simulink model "Flyback"  (R2018a)
settings: Solver=FixedStepDiscrete  StartTime=0.0  StopTime=stop_time  FixedStep=step_size  RelTol=1e-3
values from neighbouring files (symbols this model uses):
  Cf = 1e-4    (= 0.0001)    [sim_flyback.m]
  D = 0.4    [sim_flyback.m]
  f_s = 2e5    (= 200000)    [sim_flyback.m]
  R_L = 50    [sim_flyback.m]
  step_size = 1e-7    (= 1e-07)    [sim_flyback.m]
  Vd = 48    [sim_flyback.m]
libraries: powerlib x10, dspstat3 x3
settings Model: Creator=enes_  LastModifiedBy=enes_

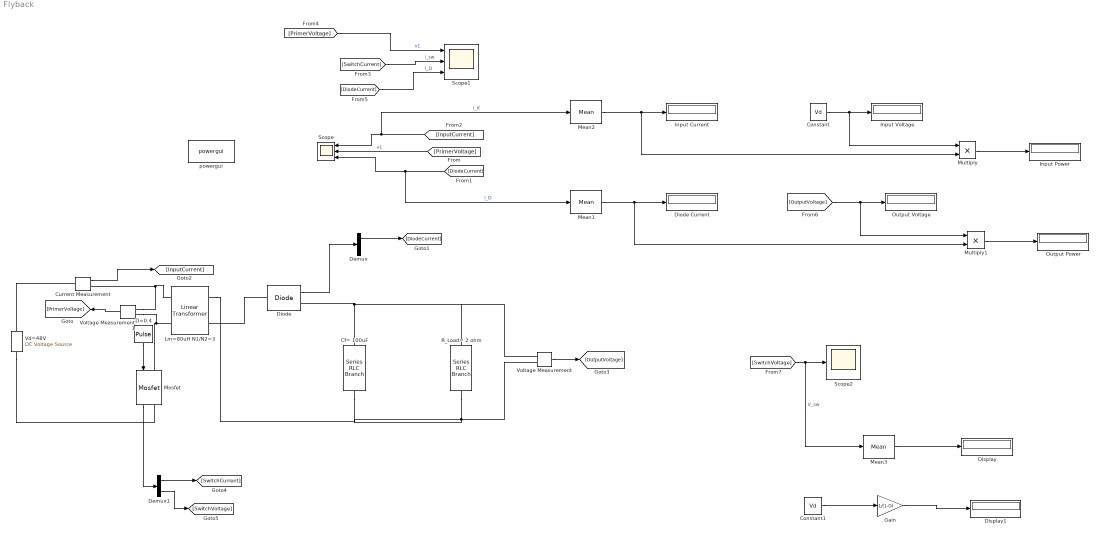
== system Flyback ==
  Cf= 100uF : powerlib/Elements/Series RLC Branch  LConnTagsString=__new0  RConnTagsString=__new0  BranchType=C  Resistance=1  Inductance=1e-3  SetiL0=off  InitialCurrent=0  Capacitance=Cf  Setx0=off  InitialVoltage=0  Measurements=None
  Constant : Constant  Value=Vd
  Constant1 : Constant  Value=Vd
  Current Measurement : powerlib/Measurements/Current Measurement  PhasorSimulation=off  OutputType=Complex  PSBequivalent=0
  D=0.4 : DiscretePulseGenerator  PulseType=Time based  Period=1/f_s  PulseWidth=100*D
  Demux : Demux  Outputs=2
  Demux1 : Demux  Outputs=2
  Diode : powerlib/Power Electronics/Diode  Ron=1e-8  Lon=0  Vf=0  IC=0  UseSnubber=0  Rs=500  Cs=250e-9  Measurements=on
  Diode Current : Display
  Display : Display
  Display1 : Display
  Gain : Gain  Gain=1/(1-D)
  Input Current : Display
  Input Power : Display
  Input Voltage : Display
  Lm=80uH N1/N2=3 : powerlib/Elements/Linear Transformer  UNITS=SI  NominalPower=[ 25 2e5 ]  winding1=[48 1e-8 1e-8 ]  winding2=[16 1e-8 1e-8]  ThreeWindings=off  winding3=[3.15e+05 0.7938 0.084225]  RmLm=[1e9 8e-5]  Measurements=All voltages and currents  DataType=on
  Mean1 : dspstat3/Mean  run=on  InputProcessing=Columns as channels (frame based)  reset_popup=None  directionMode=Each column  dimension=1  roiEnable=off  roiType=Rectangles  roiPortion=Entire ROI  roiOutput=Individual statistics for each ROI  roiFlag=off  roundingMode=Floor  overflowMode=off  outputDataTypeStr=Inherit: Same as accumulator  outputMin=[]  outputMax=[]  outputLastDataTypeStr=Inherit: Same as accumulator
  Mean2 : dspstat3/Mean  run=on  InputProcessing=Columns as channels (frame based)  reset_popup=None  directionMode=Each column  dimension=1  roiEnable=off  roiType=Rectangles  roiPortion=Entire ROI  roiOutput=Individual statistics for each ROI  roiFlag=off  roundingMode=Floor  overflowMode=off  outputDataTypeStr=Inherit: Same as accumulator  outputMin=[]  outputMax=[]  outputLastDataTypeStr=Inherit: Same as accumulator
  Mean3 : dspstat3/Mean  run=on  InputProcessing=Columns as channels (frame based)  reset_popup=None  directionMode=Each column  dimension=1  roiEnable=off  roiType=Rectangles  roiPortion=Entire ROI  roiOutput=Individual statistics for each ROI  roiFlag=off  roundingMode=Floor  overflowMode=off  outputDataTypeStr=Inherit: Same as accumulator  outputMin=[]  outputMax=[]  outputLastDataTypeStr=Inherit: Same as accumulator
  Mosfet : powerlib/Power Electronics/Mosfet  Ron=1e-8  Lon=0  Rd=1e-8  Vfd=0  IC=0  Rs=1e5  Cs=inf  Measurements=on
  Multiply : Product
  Multiply1 : Product
  Output Power : Display
  Output Voltage : Display
  R_Load= 2 ohm : powerlib/Elements/Series RLC Branch  LConnTagsString=__new0  RConnTagsString=__new0  BranchType=R  Resistance=R_L  Inductance=1e-3  SetiL0=off  InitialCurrent=0  Capacitance=Cf  Setx0=off  InitialVoltage=0  Measurements=None
  Scope : Scope  NumInputPorts=3
  Scope1 : Scope  NumInputPorts=3
  Scope2 : Scope
  Vd=48V : powerlib/Electrical Sources/DC Voltage Source  Amplitude=Vd  Measurements=None
  Voltage Measurement : powerlib/Measurements/Voltage Measurement  PhasorSimulation=off  OutputType=Complex  PSBequivalent=0
  Voltage Measurement1 : powerlib/Measurements/Voltage Measurement  PhasorSimulation=off  OutputType=Complex  PSBequivalent=0
  powergui : powerlib/powergui  Priority=1  SimulationMode=Discrete  SampleTime=step_size  frequency=60  Iterations=50  frequencyindice=0  Pbase=100e6  ErrMax=1e-4  UnitsV=kV  UnitsW=MW  buscounter=0  FunctionMessages=off  echomessages=off  EnableUseOfTLC=off  CurrentSourceSwitches=off  DisableSnubberDevices=off  DisableRonSwitches=off  DisableVfSwitches=off  DisplayEquations=off  SolverType=Tustin/Backward Euler (TBE)  Interpol=off  ExternalGateDelay=off  methode=off  Ts=100  x0status=blocks  SPID=on  SwTol=0  HookPort=off  RestoreLinks=warning  ResistiveCurrentMeasurement=off  Frange=[0:2:500]  Ylog=off  Xlog=on  ShowGrid=off  save=off  variable=ZData  structure=0  ZoomFFT=off  StartTime=0.0  cycles=1  DisplayStyle=1  fundamental=60  FreqAxis=off  MaxFrequency=1000  frequencyindicesteady=1  RmsSteady=1  display=off
  wires:
  D=0.4/1 -> Mosfet/1
  Voltage Measurement1/1 -> [PrimerVoltage]
  Diode/1 -> Demux/1
  Demux/1 -> [DiodeCurrent]
  Current Measurement/1 -> [InputCurrent]
  [InputCurrent] -> Mean2/1, Scope/1  "i_d"
  [PrimerVoltage] -> Scope/2  "v1"
  [DiodeCurrent] -> Mean1/1, Scope/3  "i_D"
  Voltage Measurement/1 -> [OutputVoltage]
  Mosfet/1 -> Demux1/1
  Demux1/1 -> [SwitchCurrent]
  [PrimerVoltage] -> Scope1/1  "v1"
  [SwitchCurrent] -> Scope1/2  "i_sw"
  [DiodeCurrent] -> Scope1/3  "i_D"
  Mean2/1 -> Multiply/2, Input Current/1
  Mean1/1 -> Multiply1/2, Diode Current/1
  [OutputVoltage] -> Multiply1/1, Output Voltage/1
  Constant/1 -> Multiply/1, Input Voltage/1
  Multiply/1 -> Input Power/1
  Multiply1/1 -> Output Power/1
  Demux1/2 -> [SwitchVoltage]
  [SwitchVoltage] -> Mean3/1, Scope2/1  "V_sw"
  Constant1/1 -> Gain/1
  Mean3/1 -> Display/1
  Gain/1 -> Display1/1
  connections:
  Voltage Measurement1/LConn1 -- Current Measurement/RConn1 -- Lm=80uH N1/N2=3/LConn1
  Mosfet/LConn1 -- Voltage Measurement1/LConn2 -- Lm=80uH N1/N2=3/LConn2
  Vd=48V/LConn1 -- Mosfet/RConn1
  Cf= 100uF/LConn1 -- Voltage Measurement/LConn1 -- R_Load= 2 ohm/LConn1 -- Diode/RConn1
  Voltage Measurement/LConn2 -- Lm=80uH N1/N2=3/RConn1 -- Cf= 100uF/RConn1 -- R_Load= 2 ohm/RConn1
  Diode/LConn1 -- Lm=80uH N1/N2=3/RConn2
  Current Measurement/LConn1 -- Vd=48V/RConn1
